simulink model "CM010C_GmG2kcaMcuCfg"  (R2013b)
settings: Solver=FixedStepDiscrete  SolverMode=SingleTasking  StartTime=0.0  StopTime=1  FixedStep=0.0005  RelTol=1e-3
values from neighbouring files (symbols this model uses):
  BATTVLTGSCAGFAC_ULS_F32 = DataDict.Constant    [CM010C_GmG2kcaMcuCfg_DataDict.m]
  BATTVLTGSWD1SCAGFAC_ULS_F32 = DataDict.Constant    [CM010C_GmG2kcaMcuCfg_DataDict.m]
undefined symbols (not defined in the file or in its folder): sigbuilder_block
libraries: CM010C_GmG2kcaMcuCfg_ModelLibrary x48, simulink x32
(part 1 of 2)
settings Model: Creator=nz3zln  LastModifiedBy=nz3zln
settings SolverCC: AutoInsertRateTranBlk=on  InsertRTBMode=Always
settings DataIOCC: LimitDataPoints=off  SaveFormat=Structure  ReturnWorkspaceOutputs=on
settings OptimizationCC: BlockReduction=off  InlineParams=on  ZeroExternalMemoryAtStartup=off  ZeroInternalMemoryAtStartup=off  OptimizeModelRefInitCode=on  LifeSpan=1
settings DebuggingCC: SignalInfNanChecking=error  SignalRangeChecking=warning  UnderspecifiedInitializationDetection=Simplified  SolverPrmCheckMsg=error  InheritedTsInSrcMsg=error  DiscreteInheritContinuousMsg=error  SingleTaskRateTransMsg=error  TasksWithSamePriorityMsg=error  SigSpecEnsureSampleTimeMsg=error  CheckMatrixSingularityMsg=error  ParameterUnderflowMsg=error  ParameterPrecisionLossMsg=error  ParameterTunabilityLossMsg=error  FixptConstUnderflowMsg=warning  FixptConstOverflowMsg=warning  VectorMatrixConversionMsg=error  SignalLabelMismatchMsg=error  UnconnectedInputMsg=error  UnconnectedOutputMsg=error  UnconnectedLineMsg=error  SFcnCompatibilityMsg=error  UniqueDataStoreMsg=warning  BusObjectLabelMismatch=error  RootOutportRequireBusObject=error  AssertControl=DisableAll  ModelReferenceIOMsg=error  ModelReferenceVersionMismatchMessage=warning  ModelReferenceIOMismatchMessage=error  ModelReferenceCSMismatchMessage=warning  ModelReferenceDataLoggingMessage=error  StateNameClashWarn=warning  StrictBusMsg=ErrorOnBusTreatedAsVector  NonBusSignalsTreatedAsBus=error  SFUnexpectedBacktrackingDiag=error  SFInvalidInputDataAccessInChartInitDiag=error  SFNoUnconditionalDefaultTransitionDiag=error  SFTransitionOutsideNaturalParentDiag=error  SFUnconditionalTransitionShadowingDiag=error  SFUndirectedBroadcastEventsDiag=error
settings ModelReferenceCC: ModelReferenceNumInstancesAllowed=Single
settings RTWCC: SystemTargetFile=autosar.tlc  GenCodeOnly=on  TemplateMakefile=ert_default_tmf  Description=AUTOSAR  GenerateReport=on  ProcessScript=autosar_make_rtw_hook  LaunchReport=on
settings CodeAppCC: GenerateComments=off  IgnoreCustomStorageClasses=off  CustomSymbolStrType=$N$R$M  CustomSymbolStrBlkIO=$N$M  SimulinkBlockComments=off
settings STFCustomTargetCC: ParMdlRefBuildCompliant=on  CompOptLevelCompliant=on  IncludeMdlTerminateFcn=off  CombineOutputUpdateFcns=on  SuppressErrorStatus=on  ERTFirstTimeCompliant=on  ERTCustomFileBanners=on  SupportNonFinite=off  SupportComplex=off  SupportContinuousTime=off  SupportNonInlinedSFcns=off  MATLABClassNameForMDSCustomization=Simulink.SoftwareTarget.ERTCustomization  AutosarCompliant=on  GRTInterface=off  SystemTargetFile=autosar.tlc
settings ERTTargetCC: CodeReplacementLibrary=ANSI_C  ConcurrentExecutionCompliant=off  IncludeMdlTerminateFcn=off  SuppressErrorStatus=on  SupportNonFinite=off  SupportComplex=off  ModelStepFunctionPrototypeControlCompliant=off  CPPClassGenCompliant=off  AutosarCompliant=on  InlinedParameterPlacement=NonHierarchical  ERTCustomFileTemplate=example_file_process.tlc  EnableUserReplacementTypes=on

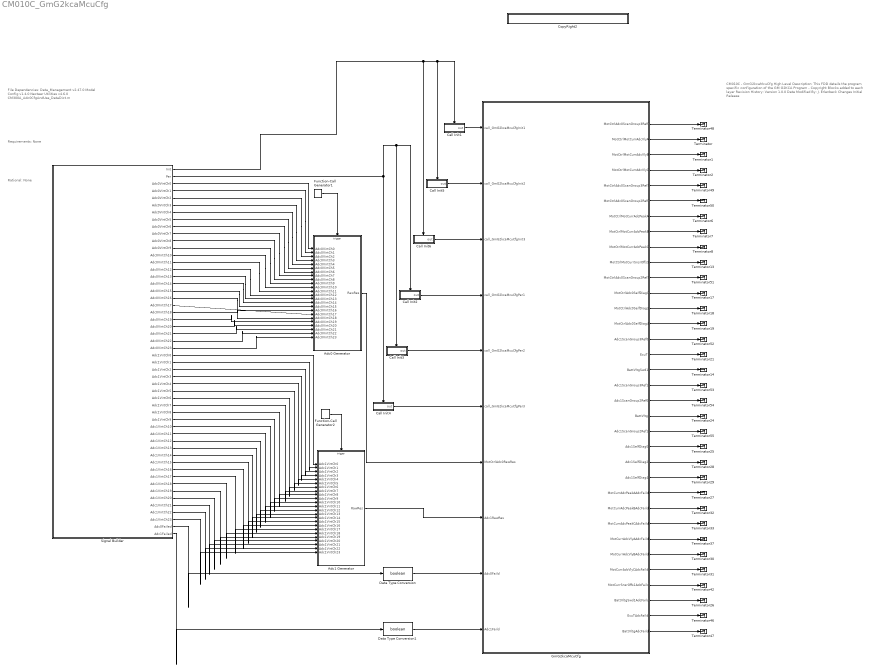
== system CM010C_GmG2kcaMcuCfg ==
  note: File Dependencies:
      |
      | Data_Management v2.47.0
      | Model Config v1.4.0
      | Nexteer Utilities v4.6.0
      | CM300A_Adc0CfgAndUse_DataDict.m
  note: CM010C - GmG2kcaMcuCfg
      |
      | High Level Description:
      | This FDD details the program specific configuration of the GM G2KCA Program
      |  - Copyright Blocks added to each layer
      |
      | Revision History:
      |
      | Version		1.0.0
      | Date
      | Modified By: 	J. Erlenbeck
      | Changes		Initial Release
  note: Requirements:
      |
      | None
  note: Rational:
      |
      | None
  Adc0 Generator : Subsystem  TreatAsAtomicUnit=on
  Adc1 Generator : Subsystem  TreatAsAtomicUnit=on
  Call Init1 : Subsystem  TreatAsAtomicUnit=on
  Call Init2 : Subsystem  TreatAsAtomicUnit=on
  Call Init3 : Subsystem  TreatAsAtomicUnit=on
  Call Init4 : Subsystem  TreatAsAtomicUnit=on
  Call Init5 : Subsystem  TreatAsAtomicUnit=on
  Call Init6 : Subsystem  TreatAsAtomicUnit=on
  CopyRight2 : Subsystem  Description=|  mask(Copyright Information){none=on}
      | Copyright info block.                                               
      |                                                                     
      | Place copyright information at the top of every subsystem in design.
      mask prompts: none "No parameters"
      mask help: Place copyright information at the top of every subsystem in design.
      mask Display:
      | NxtrConf = 'Nexteer Confidential';
      | 
      | sys = bdroot; %handle for the current model ("system")
      | first = get_param(sys,'Created');
      | first = first(end-3:end);  %year is last four digits
      | 
      | last = get_param(sys,'LastModifiedDate');
      | if isempty(last)
      |     last = datestr(now,'yyyy');
      | else
      |     last = last(end-3:end);
      | end
      | 
      | if strcmp(first,last)
      |     fprintf('%s -- Copyright %s Nexteer',NxtrConf,first)
      | else
      |     fprintf('%s -- %s%s- %s Nexteer',NxtrConf,char(169),first,last)
      | end
  Data Type Conversion : DataTypeConversion  OutDataTypeStr=boolean
  Data Type Conversion1 : DataTypeConversion  OutDataTypeStr=boolean
  Function-Call Generator1 : simulink/Ports & Subsystems/Function-Call Generator  sample_time=0.0005  numberOfIterations=1
  Function-Call Generator2 : simulink/Ports & Subsystems/Function-Call Generator  sample_time=0.0005  numberOfIterations=1
  GmG2kcaMcuCfg : Subsystem
  Signal Builder : Subsystem  Tag=STV Subsys  RequirementInfo={} %GIDa_2822100e_29fa_4197_9ccc_01864625f252  LoadFcn=sigbuilder_block('load');  StartFcn=sigbuilder_block('start');  StopFcn=sigbuilder_block('stop');  ClipboardFcn=sigbuilder_block('clipboard');  mask(Sigbuilder block){}
      mask help: Simulink:masks:SigbuilderBlock_MD
      mask init:
      | if ~strcmp(get_param(bdroot(gcbh),'SimulationStatus'),'stopped') tuvar = sigbuilder_block('maskInit'); end
      settings: CopyFcn=sigbuilder_block('copy');  DeleteFcn=sigbuilder_block('delete');  ModelCloseFcn=sigbuilder_block('modelClose');  PreSaveFcn=sigbuilder_block('preSave');  PauseFcn=sigbuilder_block('pause');  ContinueFcn=sigbuilder_block('continue');  NameChangeFcn=sigbuilder_block('namechange');  OpenFcn=sigbuilder_block('open',[6.2069 35.3793 1178.69 576 ]);  CloseFcn=sigbuilder_block('close');
      mask Display: plot(0, 0, 100, 100,[2, 2, 32, 32, 2], [68, 8, 8, 68, 68],[32, 2], [38, 38], [32, 19, 2],[53, 60, 44], [32, 17, 17, 2],[16, 16, 31, 31]);txt = getActiveGroup(gcbh);text(2, 100, txt,'verticalAlignment', 'top');
  Terminator{,1..2,6..8,13..14,17..19,21,24..33,37,42,46..55} (34 alike) : Terminator
  wires:
  Call Init1/1(out) -> GmG2kcaMcuCfg/1(call_GmG2kcaMcuCfgInit1)
  Call Init2/1(out) -> GmG2kcaMcuCfg/4(call_GmG2kcaMcuCfgPer1)
  Call Init3/1(out) -> GmG2kcaMcuCfg/5(call_GmG2kcaMcuCfgPer2)
  GmG2kcaMcuCfg/2(MotCtrlMotCurrAdcVlyA) -> Terminator/1
  GmG2kcaMcuCfg/3(MotCtrlMotCurrAdcVlyB) -> Terminator1/1
  GmG2kcaMcuCfg/4(MotCtrlMotCurrAdcVlyC) -> Terminator2/1
  GmG2kcaMcuCfg/7(MotCtrlMotCurrAdcPeakA) -> Terminator6/1
  GmG2kcaMcuCfg/8(MotCtrlMotCurrAdcPeakB) -> Terminator7/1
  GmG2kcaMcuCfg/9(MotCtrlMotCurrAdcPeakC) -> Terminator8/1
  GmG2kcaMcuCfg/10(MotCtrlMotCurrSnsrOffs1) -> Terminator13/1
  GmG2kcaMcuCfg/12(MotCtrlAdc0SelfDiag0) -> Terminator17/1
  GmG2kcaMcuCfg/13(MotCtrlAdc0SelfDiag2) -> Terminator18/1
  GmG2kcaMcuCfg/14(MotCtrlAdc0SelfDiag4) -> Terminator19/1
  GmG2kcaMcuCfg/16(EcuT) -> Terminator21/1
  GmG2kcaMcuCfg/17(BattVltgSwd1) -> Terminator14/1
  GmG2kcaMcuCfg/20(BattVltg) -> Terminator24/1
  GmG2kcaMcuCfg/22(Adc1SelfDiag0) -> Terminator25/1
  GmG2kcaMcuCfg/23(Adc1SelfDiag2) -> Terminator28/1
  GmG2kcaMcuCfg/24(Adc1SelfDiag4) -> Terminator29/1
  GmG2kcaMcuCfg/25(MotCurrAdcPeakAAdcFaild) -> Terminator27/1
  GmG2kcaMcuCfg/26(MotCurrAdcPeakBAdcFaild) -> Terminator32/1
  GmG2kcaMcuCfg/27(MotCurrAdcPeakCAdcFaild) -> Terminator33/1
  GmG2kcaMcuCfg/28(MotCurrAdcVlyAAdcFaild) -> Terminator37/1
  GmG2kcaMcuCfg/29(MotCurrAdcVlyBAdcFaild) -> Terminator30/1
  GmG2kcaMcuCfg/30(MotCurrAdcVlyCAdcFaild) -> Terminator31/1
  GmG2kcaMcuCfg/31(MotCurrSnsrOffs1AdcFaild) -> Terminator42/1
  GmG2kcaMcuCfg/32(BattVltgSwd1AdcFaild) -> Terminator26/1
  GmG2kcaMcuCfg/33(EcuTAdcFaild) -> Terminator46/1
  Call Init4/1(out) -> GmG2kcaMcuCfg/6(call_GmG2kcaMcuCfgPer3)
  Call Init5/1(out) -> GmG2kcaMcuCfg/2(call_GmG2kcaMcuCfgInit2)
  Call Init6/1(out) -> GmG2kcaMcuCfg/3(call_GmG2kcaMcuCfgInit3)
  GmG2kcaMcuCfg/34(BattVltgAdcFaild) -> Terminator47/1
  GmG2kcaMcuCfg/1(MotCtrlAdc0ScanGroup3Ref0) -> Terminator48/1
  GmG2kcaMcuCfg/5(MotCtrlAdc0ScanGroup3Ref1) -> Terminator49/1
  GmG2kcaMcuCfg/6(MotCtrlAdc0ScanGroup2Ref0) -> Terminator50/1
  GmG2kcaMcuCfg/11(MotCtrlAdc0ScanGroup2Ref1) -> Terminator51/1
  GmG2kcaMcuCfg/15(Adc1ScanGroup3Ref0) -> Terminator52/1
  GmG2kcaMcuCfg/18(Adc1ScanGroup3Ref1) -> Terminator53/1
  GmG2kcaMcuCfg/19(Adc1ScanGroup2Ref0) -> Terminator54/1
  GmG2kcaMcuCfg/21(Adc1ScanGroup2Ref1) -> Terminator55/1
  Function-Call Generator1/1 -> Adc0 Generator/Trigger
  Signal Builder/1(Init) -> Call Init6/Enable, Call Init5/Enable, Call Init1/Enable
  Signal Builder/2(Per) -> Call Init3/Enable, Call Init2/Enable, Call Init4/Enable
  Signal Builder/26(Adc0VirtCh23) -> Adc0 Generator/24(Adc0VirtCh23)
  Signal Builder/25(Adc0VirtCh22) -> Adc0 Generator/23(Adc0VirtCh22)
  Signal Builder/24(Adc0VirtCh21) -> Adc0 Generator/22(Adc0VirtCh21)
  Signal Builder/23(Adc0VirtCh20) -> Adc0 Generator/21(Adc0VirtCh20)
  Signal Builder/22(Adc0VirtCh19) -> Adc0 Generator/20(Adc0VirtCh19)
  Signal Builder/21(Adc0VirtCh18) -> Adc0 Generator/19(Adc0VirtCh18)
  Signal Builder/20(Adc0VirtCh17) -> Adc0 Generator/18(Adc0VirtCh17)
  Signal Builder/19(Adc0VirtCh16) -> Adc0 Generator/17(Adc0VirtCh16)
  Signal Builder/18(Adc0VirtCh15) -> Adc0 Generator/16(Adc0VirtCh15)
  Signal Builder/17(Adc0VirtCh14) -> Adc0 Generator/15(Adc0VirtCh14)
  Signal Builder/16(Adc0VirtCh13) -> Adc0 Generator/14(Adc0VirtCh13)
  Signal Builder/15(Adc0VirtCh12) -> Adc0 Generator/13(Adc0VirtCh12)
  Signal Builder/14(Adc0VirtCh11) -> Adc0 Generator/12(Adc0VirtCh11)
  Signal Builder/13(Adc0VirtCh10) -> Adc0 Generator/11(Adc0VirtCh10)
  Signal Builder/12(Adc0VirtCh9) -> Adc0 Generator/10(Adc0VirtCh9)
  Signal Builder/11(Adc0VirtCh8) -> Adc0 Generator/9(Adc0VirtCh8)
  Signal Builder/10(Adc0VirtCh7) -> Adc0 Generator/8(Adc0VirtCh7)
  Signal Builder/9(Adc0VirtCh6) -> Adc0 Generator/7(Adc0VirtCh6)
  Signal Builder/8(Adc0VirtCh5) -> Adc0 Generator/6(Adc0VirtCh5)
  Signal Builder/7(Adc0VirtCh4) -> Adc0 Generator/5(Adc0VirtCh4)
  Signal Builder/6(Adc0VirtCh3) -> Adc0 Generator/4(Adc0VirtCh3)
  Signal Builder/5(Adc0VirtCh2) -> Adc0 Generator/3(Adc0VirtCh2)
  Signal Builder/4(Adc0VirtCh1) -> Adc0 Generator/2(Adc0VirtCh1)
  Signal Builder/3(Adc0VirtCh0) -> Adc0 Generator/1(Adc0VirtCh0)
  Adc0 Generator/1(RawRes) -> GmG2kcaMcuCfg/7(MotCtrlAdc0RawRes)
  Signal Builder/50(Adc1VirtCh23) -> Adc1 Generator/24(Adc1VirtCh23)
  Signal Builder/49(Adc1VirtCh22) -> Adc1 Generator/23(Adc1VirtCh22)
  Signal Builder/48(Adc1VirtCh21) -> Adc1 Generator/22(Adc1VirtCh21)
  Signal Builder/47(Adc1VirtCh20) -> Adc1 Generator/21(Adc1VirtCh20)
  Signal Builder/46(Adc1VirtCh19) -> Adc1 Generator/20(Adc1VirtCh19)
  Signal Builder/45(Adc1VirtCh18) -> Adc1 Generator/19(Adc1VirtCh18)
  Signal Builder/44(Adc1VirtCh17) -> Adc1 Generator/18(Adc1VirtCh17)
  Signal Builder/43(Adc1VirtCh16) -> Adc1 Generator/17(Adc1VirtCh16)
  Signal Builder/42(Adc1VirtCh15) -> Adc1 Generator/16(Adc1VirtCh15)
  Signal Builder/41(Adc1VirtCh14) -> Adc1 Generator/15(Adc1VirtCh14)
  Signal Builder/40(Adc1VirtCh13) -> Adc1 Generator/14(Adc1VirtCh13)
  Signal Builder/39(Adc1VirtCh12) -> Adc1 Generator/13(Adc1VirtCh12)
  Signal Builder/38(Adc1VirtCh11) -> Adc1 Generator/12(Adc1VirtCh11)
  Signal Builder/37(Adc1VirtCh10) -> Adc1 Generator/11(Adc1VirtCh10)
  Signal Builder/36(Adc1VirtCh9) -> Adc1 Generator/10(Adc1VirtCh9)
  Signal Builder/35(Adc1VirtCh8) -> Adc1 Generator/9(Adc1VirtCh8)
  Signal Builder/34(Adc1VirtCh7) -> Adc1 Generator/8(Adc1VirtCh7)
  Signal Builder/33(Adc1VirtCh6) -> Adc1 Generator/7(Adc1VirtCh6)
  Signal Builder/32(Adc1VirtCh5) -> Adc1 Generator/6(Adc1VirtCh5)
  Signal Builder/31(Adc1VirtCh4) -> Adc1 Generator/5(Adc1VirtCh4)
  Signal Builder/30(Adc1VirtCh3) -> Adc1 Generator/4(Adc1VirtCh3)
  Signal Builder/29(Adc1VirtCh2) -> Adc1 Generator/3(Adc1VirtCh2)
  Signal Builder/28(Adc1VirtCh1) -> Adc1 Generator/2(Adc1VirtCh1)
  Signal Builder/27(Adc1VirtCh0) -> Adc1 Generator/1(Adc1VirtCh0)
  Function-Call Generator2/1 -> Adc1 Generator/Trigger
  Adc1 Generator/1(RawRes) -> GmG2kcaMcuCfg/8(Adc1RawRes)
  Signal Builder/51(Adc0Failed) -> Data Type Conversion/1
  Signal Builder/52(Adc1Failed) -> Data Type Conversion1/1
  Data Type Conversion/1 -> GmG2kcaMcuCfg/9(Adc0Faild)
  Data Type Conversion1/1 -> GmG2kcaMcuCfg/10(Adc1Faild)

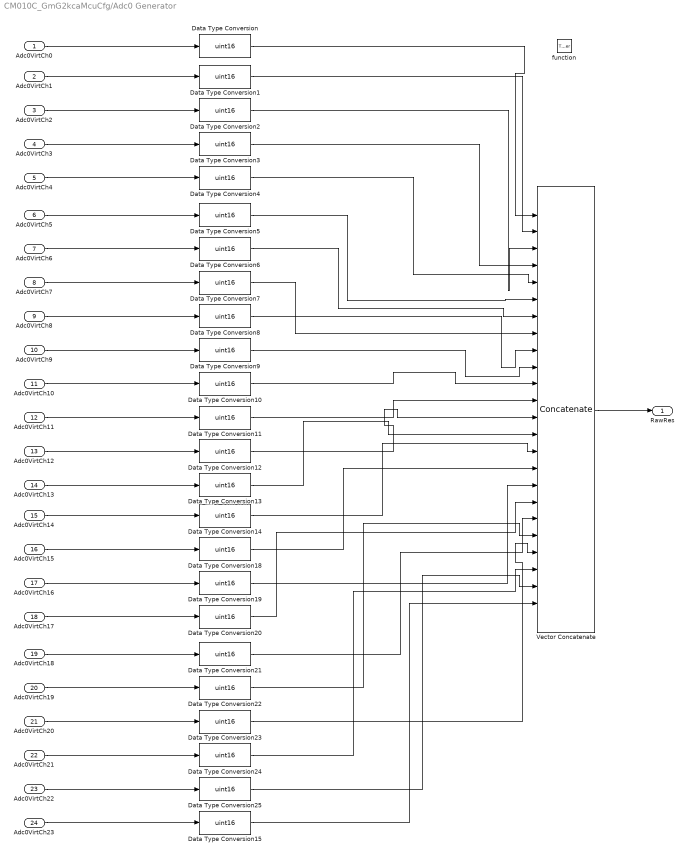
== system CM010C_GmG2kcaMcuCfg/Adc0 Generator ==
  Adc0VirtCh0 : Inport
  Adc0VirtCh1 : Inport  Port=2
  Adc0VirtCh2 : Inport  Port=3
  Adc0VirtCh3 : Inport  Port=4
  Adc0VirtCh4 : Inport  Port=5
  Adc0VirtCh5 : Inport  Port=6
  Adc0VirtCh6 : Inport  Port=7
  Adc0VirtCh7 : Inport  Port=8
  Adc0VirtCh8 : Inport  Port=9
  Adc0VirtCh9 : Inport  Port=10
  Adc0VirtCh10 : Inport  Port=11
  Adc0VirtCh11 : Inport  Port=12
  Adc0VirtCh12 : Inport  Port=13
  Adc0VirtCh13 : Inport  Port=14
  Adc0VirtCh14 : Inport  Port=15
  Adc0VirtCh15 : Inport  Port=16
  Adc0VirtCh16 : Inport  Port=17
  Adc0VirtCh17 : Inport  Port=18
  Adc0VirtCh18 : Inport  Port=19
  Adc0VirtCh19 : Inport  Port=20
  Adc0VirtCh20 : Inport  Port=21
  Adc0VirtCh21 : Inport  Port=22
  Adc0VirtCh22 : Inport  Port=23
  Adc0VirtCh23 : Inport  Port=24
  function : TriggerPort  TriggerType=function-call
  Data Type Conversion{,1..15,18..25} (24 alike) : DataTypeConversion  OutDataTypeStr=uint16
  Vector Concatenate : Concatenate  NumInputs=24
  RawRes : Outport
  wires:
  Adc0VirtCh0/1 -> Data Type Conversion/1
  Data Type Conversion/1 -> Vector Concatenate/1
  Adc0VirtCh1/1 -> Data Type Conversion1/1
  Adc0VirtCh2/1 -> Data Type Conversion2/1
  Adc0VirtCh3/1 -> Data Type Conversion3/1
  Adc0VirtCh4/1 -> Data Type Conversion4/1
  Adc0VirtCh5/1 -> Data Type Conversion5/1
  Adc0VirtCh6/1 -> Data Type Conversion6/1
  Adc0VirtCh7/1 -> Data Type Conversion7/1
  Adc0VirtCh8/1 -> Data Type Conversion8/1
  Adc0VirtCh9/1 -> Data Type Conversion9/1
  Adc0VirtCh10/1 -> Data Type Conversion10/1
  Adc0VirtCh11/1 -> Data Type Conversion11/1
  Adc0VirtCh12/1 -> Data Type Conversion12/1
  Adc0VirtCh13/1 -> Data Type Conversion13/1
  Adc0VirtCh14/1 -> Data Type Conversion14/1
  Adc0VirtCh15/1 -> Data Type Conversion18/1
  Adc0VirtCh17/1 -> Data Type Conversion20/1
  Adc0VirtCh18/1 -> Data Type Conversion21/1
  Adc0VirtCh19/1 -> Data Type Conversion22/1
  Adc0VirtCh20/1 -> Data Type Conversion23/1
  Adc0VirtCh21/1 -> Data Type Conversion24/1
  Adc0VirtCh23/1 -> Data Type Conversion15/1
  Adc0VirtCh16/1 -> Data Type Conversion19/1
  Adc0VirtCh22/1 -> Data Type Conversion25/1
  Data Type Conversion1/1 -> Vector Concatenate/2
  Data Type Conversion2/1 -> Vector Concatenate/3
  Data Type Conversion3/1 -> Vector Concatenate/4
  Data Type Conversion4/1 -> Vector Concatenate/5
  Data Type Conversion5/1 -> Vector Concatenate/6
  Data Type Conversion6/1 -> Vector Concatenate/7
  Data Type Conversion7/1 -> Vector Concatenate/8
  Data Type Conversion8/1 -> Vector Concatenate/9
  Data Type Conversion9/1 -> Vector Concatenate/10
  Data Type Conversion10/1 -> Vector Concatenate/11
  Data Type Conversion11/1 -> Vector Concatenate/12
  Data Type Conversion12/1 -> Vector Concatenate/13
  Data Type Conversion13/1 -> Vector Concatenate/14
  Data Type Conversion14/1 -> Vector Concatenate/15
  Data Type Conversion18/1 -> Vector Concatenate/16
  Data Type Conversion19/1 -> Vector Concatenate/17
  Data Type Conversion20/1 -> Vector Concatenate/18
  Data Type Conversion21/1 -> Vector Concatenate/19
  Data Type Conversion22/1 -> Vector Concatenate/20
  Data Type Conversion23/1 -> Vector Concatenate/21
  Data Type Conversion24/1 -> Vector Concatenate/22
  Data Type Conversion25/1 -> Vector Concatenate/23
  Data Type Conversion15/1 -> Vector Concatenate/24
  Vector Concatenate/1 -> RawRes/1

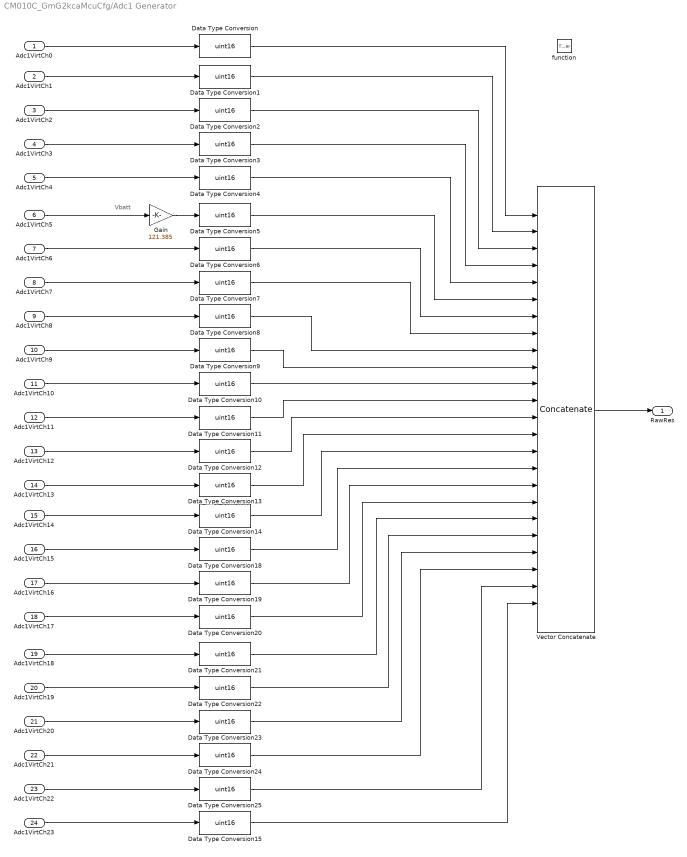
== system CM010C_GmG2kcaMcuCfg/Adc1 Generator ==
  note: Vbatt
  Adc1VirtCh0 : Inport
  Adc1VirtCh1 : Inport  Port=2
  Adc1VirtCh2 : Inport  Port=3
  Adc1VirtCh3 : Inport  Port=4
  Adc1VirtCh4 : Inport  Port=5
  Adc1VirtCh5 : Inport  Port=6
  Adc1VirtCh6 : Inport  Port=7
  Adc1VirtCh7 : Inport  Port=8
  Adc1VirtCh8 : Inport  Port=9
  Adc1VirtCh9 : Inport  Port=10
  Adc1VirtCh10 : Inport  Port=11
  Adc1VirtCh11 : Inport  Port=12
  Adc1VirtCh12 : Inport  Port=13
  Adc1VirtCh13 : Inport  Port=14
  Adc1VirtCh14 : Inport  Port=15
  Adc1VirtCh15 : Inport  Port=16
  Adc1VirtCh16 : Inport  Port=17
  Adc1VirtCh17 : Inport  Port=18
  Adc1VirtCh18 : Inport  Port=19
  Adc1VirtCh19 : Inport  Port=20
  Adc1VirtCh20 : Inport  Port=21
  Adc1VirtCh21 : Inport  Port=22
  Adc1VirtCh22 : Inport  Port=23
  Adc1VirtCh23 : Inport  Port=24
  function : TriggerPort  TriggerType=function-call
  Data Type Conversion{,1..15,18..25} (24 alike) : DataTypeConversion  OutDataTypeStr=uint16
  Gain : Gain  Gain=121.385
  Vector Concatenate : Concatenate  NumInputs=24
  RawRes : Outport
  wires:
  Vector Concatenate/1 -> RawRes/1
  Data Type Conversion15/1 -> Vector Concatenate/24
  Data Type Conversion25/1 -> Vector Concatenate/23
  Data Type Conversion24/1 -> Vector Concatenate/22
  Data Type Conversion23/1 -> Vector Concatenate/21
  Data Type Conversion22/1 -> Vector Concatenate/20
  Data Type Conversion21/1 -> Vector Concatenate/19
  Data Type Conversion20/1 -> Vector Concatenate/18
  Data Type Conversion19/1 -> Vector Concatenate/17
  Data Type Conversion18/1 -> Vector Concatenate/16
  Data Type Conversion14/1 -> Vector Concatenate/15
  Data Type Conversion13/1 -> Vector Concatenate/14
  Data Type Conversion12/1 -> Vector Concatenate/13
  Data Type Conversion11/1 -> Vector Concatenate/12
  Data Type Conversion10/1 -> Vector Concatenate/11
  Data Type Conversion9/1 -> Vector Concatenate/10
  Data Type Conversion8/1 -> Vector Concatenate/9
  Data Type Conversion7/1 -> Vector Concatenate/8
  Data Type Conversion6/1 -> Vector Concatenate/7
  Data Type Conversion5/1 -> Vector Concatenate/6
  Data Type Conversion4/1 -> Vector Concatenate/5
  Data Type Conversion3/1 -> Vector Concatenate/4
  Data Type Conversion2/1 -> Vector Concatenate/3
  Data Type Conversion1/1 -> Vector Concatenate/2
  Adc1VirtCh22/1 -> Data Type Conversion25/1
  Adc1VirtCh16/1 -> Data Type Conversion19/1
  Adc1VirtCh23/1 -> Data Type Conversion15/1
  Adc1VirtCh21/1 -> Data Type Conversion24/1
  Adc1VirtCh20/1 -> Data Type Conversion23/1
  Adc1VirtCh19/1 -> Data Type Conversion22/1
  Adc1VirtCh18/1 -> Data Type Conversion21/1
  Adc1VirtCh17/1 -> Data Type Conversion20/1
  Adc1VirtCh15/1 -> Data Type Conversion18/1
  Adc1VirtCh14/1 -> Data Type Conversion14/1
  Adc1VirtCh13/1 -> Data Type Conversion13/1
  Adc1VirtCh12/1 -> Data Type Conversion12/1
  Adc1VirtCh11/1 -> Data Type Conversion11/1
  Adc1VirtCh10/1 -> Data Type Conversion10/1
  Adc1VirtCh9/1 -> Data Type Conversion9/1
  Adc1VirtCh8/1 -> Data Type Conversion8/1
  Adc1VirtCh7/1 -> Data Type Conversion7/1
  Adc1VirtCh6/1 -> Data Type Conversion6/1
  Adc1VirtCh5/1 -> Gain/1
  Adc1VirtCh4/1 -> Data Type Conversion4/1
  Adc1VirtCh3/1 -> Data Type Conversion3/1
  Adc1VirtCh2/1 -> Data Type Conversion2/1
  Adc1VirtCh1/1 -> Data Type Conversion1/1
  Data Type Conversion/1 -> Vector Concatenate/1
  Adc1VirtCh0/1 -> Data Type Conversion/1
  Gain/1 -> Data Type Conversion5/1

== system CM010C_GmG2kcaMcuCfg/Call Init1 ==
  Enable : EnablePort
  Function Call Trigger : simulink/Ports & Subsystems/Function-Call Generator  RequirementInfo="{'linktype_rmi_doors' '000089e3 (/E-STEER_New/System Specification Documents/Core Specs/Subsystem Specs/System Functions FDD/SF-46  Gross Cross Check)' '#211' 'true' '3.1-1 The GCC function shall monitor every posted output motor comm' '' ; 'linktype_rmi_doors' '000089e3 (/E-STEER_New/System Specification Documents/Core Specs/Subsystem Specs/System Functions FDD/SF-46  Gross Cross Check)' '#182' 'true' '3.2.2-1 GCC shall be executed at a 0.002 second loop time.' '' } %GIDa_ff755a2e_49d1_45f7_8591_3ce0ef475338"  sample_time=0.0005  numberOfIterations=1
  out : Outport
  wires:
  Function Call Trigger/1 -> out/1

== system CM010C_GmG2kcaMcuCfg/Call Init2 ==
  Enable : EnablePort
  Function Call Trigger : simulink/Ports & Subsystems/Function-Call Generator  RequirementInfo="{'linktype_rmi_doors' '000089e3 (/E-STEER_New/System Specification Documents/Core Specs/Subsystem Specs/System Functions FDD/SF-46  Gross Cross Check)' '#211' 'true' '3.1-1 The GCC function shall monitor every posted output motor comm' '' ; 'linktype_rmi_doors' '000089e3 (/E-STEER_New/System Specification Documents/Core Specs/Subsystem Specs/System Functions FDD/SF-46  Gross Cross Check)' '#182' 'true' '3.2.2-1 GCC shall be executed at a 0.002 second loop time.' '' } %GIDa_ba5be832_aeac_40ae_ae53_3fd25198366e"  sample_time=0.0005  numberOfIterations=1
  out : Outport
  wires:
  Function Call Trigger/1 -> out/1

== system CM010C_GmG2kcaMcuCfg/Call Init3 ==
  Enable : EnablePort
  Function Call Trigger : simulink/Ports & Subsystems/Function-Call Generator  RequirementInfo="{'linktype_rmi_doors' '000089e3 (/E-STEER_New/System Specification Documents/Core Specs/Subsystem Specs/System Functions FDD/SF-46  Gross Cross Check)' '#211' 'true' '3.1-1 The GCC function shall monitor every posted output motor comm' '' ; 'linktype_rmi_doors' '000089e3 (/E-STEER_New/System Specification Documents/Core Specs/Subsystem Specs/System Functions FDD/SF-46  Gross Cross Check)' '#182' 'true' '3.2.2-1 GCC shall be executed at a 0.002 second loop time.' '' } %GIDa_bf682727_f4b1_4f52_ae72_c6f6d8d412d7"  sample_time=0.002  numberOfIterations=1
  out : Outport
  wires:
  Function Call Trigger/1 -> out/1

== system CM010C_GmG2kcaMcuCfg/Call Init4 ==
  Enable : EnablePort
  Function Call Trigger : simulink/Ports & Subsystems/Function-Call Generator  RequirementInfo="{'linktype_rmi_doors' '000089e3 (/E-STEER_New/System Specification Documents/Core Specs/Subsystem Specs/System Functions FDD/SF-46  Gross Cross Check)' '#211' 'true' '3.1-1 The GCC function shall monitor every posted output motor comm' '' ; 'linktype_rmi_doors' '000089e3 (/E-STEER_New/System Specification Documents/Core Specs/Subsystem Specs/System Functions FDD/SF-46  Gross Cross Check)' '#182' 'true' '3.2.2-1 GCC shall be executed at a 0.002 second loop time.' '' } %GIDa_39162fcb_260a_4191_9640_bf2fa4fe87e2"  sample_time=0.002  numberOfIterations=1
  out : Outport
  wires:
  Function Call Trigger/1 -> out/1

== system CM010C_GmG2kcaMcuCfg/Call Init5 ==
  Enable : EnablePort
  Function Call Trigger : simulink/Ports & Subsystems/Function-Call Generator  RequirementInfo="{'linktype_rmi_doors' '000089e3 (/E-STEER_New/System Specification Documents/Core Specs/Subsystem Specs/System Functions FDD/SF-46  Gross Cross Check)' '#211' 'true' '3.1-1 The GCC function shall monitor every posted output motor comm' '' ; 'linktype_rmi_doors' '000089e3 (/E-STEER_New/System Specification Documents/Core Specs/Subsystem Specs/System Functions FDD/SF-46  Gross Cross Check)' '#182' 'true' '3.2.2-1 GCC shall be executed at a 0.002 second loop time.' '' } %GIDa_52b82f2d_d21e_4ccf_9b87_2b660c433421"  sample_time=0.0005  numberOfIterations=1
  out : Outport
  wires:
  Function Call Trigger/1 -> out/1

== system CM010C_GmG2kcaMcuCfg/Call Init6 ==
  Enable : EnablePort
  Function Call Trigger : simulink/Ports & Subsystems/Function-Call Generator  RequirementInfo="{'linktype_rmi_doors' '000089e3 (/E-STEER_New/System Specification Documents/Core Specs/Subsystem Specs/System Functions FDD/SF-46  Gross Cross Check)' '#211' 'true' '3.1-1 The GCC function shall monitor every posted output motor comm' '' ; 'linktype_rmi_doors' '000089e3 (/E-STEER_New/System Specification Documents/Core Specs/Subsystem Specs/System Functions FDD/SF-46  Gross Cross Check)' '#182' 'true' '3.2.2-1 GCC shall be executed at a 0.002 second loop time.' '' } %GIDa_40b20fc1_ef82_4ce8_9bb2_77ecb7477d85"  sample_time=0.002  numberOfIterations=1
  out : Outport
  wires:
  Function Call Trigger/1 -> out/1

== system CM010C_GmG2kcaMcuCfg/CopyRight2 ==

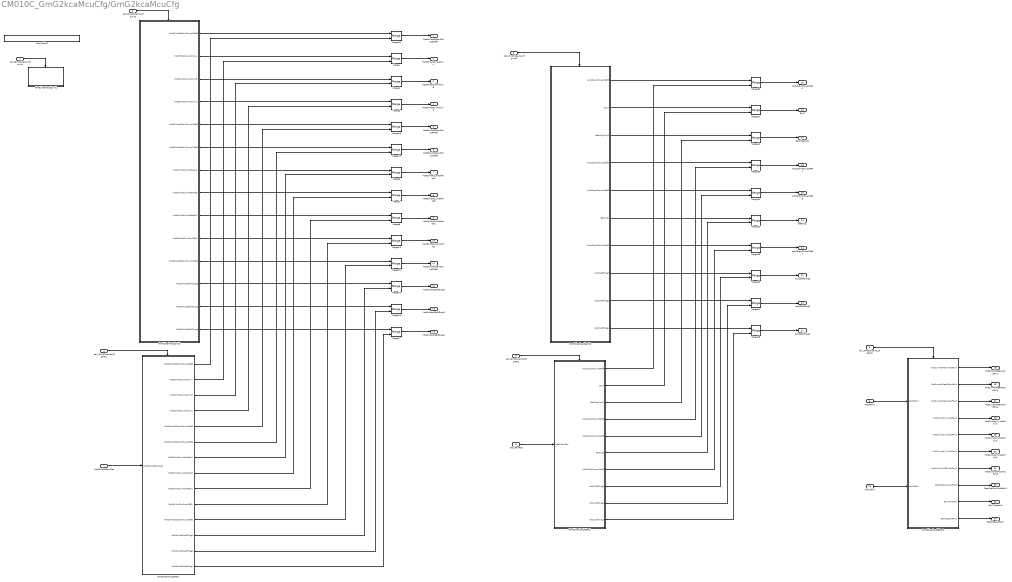
== system CM010C_GmG2kcaMcuCfg/GmG2kcaMcuCfg ==
  call_GmG2kcaMcuCfgInit1 : Inport
  call_GmG2kcaMcuCfgInit2 : Inport  Port=2
  call_GmG2kcaMcuCfgInit3 : Inport  Port=3
  call_GmG2kcaMcuCfgPer1 : Inport  Port=4
  call_GmG2kcaMcuCfgPer2 : Inport  Port=5
  call_GmG2kcaMcuCfgPer3 : Inport  Port=6
  MotCtrlAdc0RawRes : Inport  Port=7
  Adc1RawRes : Inport  Port=8
  Adc0Faild : Inport  Port=9
  Adc1Faild : Inport  Port=10
  CopyRight2 : Subsystem  Description=|  mask(Copyright Information){none=on}
      | Copyright info block.                                               
      |                                                                     
      | Place copyright information at the top of every subsystem in design.
      mask prompts: none "No parameters"
      mask help: Place copyright information at the top of every subsystem in design.
      mask Display:
      | NxtrConf = 'Nexteer Confidential';
      | 
      | sys = bdroot; %handle for the current model ("system")
      | first = get_param(sys,'Created');
      | first = first(end-3:end);  %year is last four digits
      | 
      | last = get_param(sys,'LastModifiedDate');
      | if isempty(last)
      |     last = datestr(now,'yyyy');
      | else
      |     last = last(end-3:end);
      | end
      | 
      | if strcmp(first,last)
      |     fprintf('%s -- Copyright %s Nexteer',NxtrConf,first)
      | else
      |     fprintf('%s -- %s%s- %s Nexteer',NxtrConf,char(169),first,last)
      | end
  GmG2kcaMcuCfgInit1 : Subsystem
  GmG2kcaMcuCfgInit2 : Subsystem
  GmG2kcaMcuCfgInit3 : Subsystem
  GmG2kcaMcuCfgPer1 : Subsystem  RequirementInfo={} %GIDa_cb8aed4e_f73b_4f5e_bbba_e7bbcee4a2fc
      settings: AttributesFormatString=Priority: %<Priority>
  GmG2kcaMcuCfgPer2 : Subsystem  RequirementInfo={} %GIDa_f8eec309_27b4_4df0_b18c_c2951f94362c
      settings: AttributesFormatString=Priority: %<Priority>
  GmG2kcaMcuCfgPer3 : Subsystem  RequirementInfo={} %GIDa_f61b09d0_e9f4_4379_bee3_c878705b543d
      settings: AttributesFormatString=Priority: %<Priority>
  Merge{,1..2,6..8,13,15..17,20,22..25,27..35} (24 alike) : Merge
  MotCtrlAdc0ScanGroup3Ref0 : Outport
  MotCtrlMotCurrAdcVlyA : Outport  Port=2
  MotCtrlMotCurrAdcVlyB : Outport  Port=3
  MotCtrlMotCurrAdcVlyC : Outport  Port=4
  MotCtrlAdc0ScanGroup3Ref1 : Outport  Port=5
  MotCtrlAdc0ScanGroup2Ref0 : Outport  Port=6
  MotCtrlMotCurrAdcPeakA : Outport  Port=7
  MotCtrlMotCurrAdcPeakB : Outport  Port=8
  MotCtrlMotCurrAdcPeakC : Outport  Port=9
  MotCtrlMotCurrSnsrOffs1 : Outport  Port=10
  MotCtrlAdc0ScanGroup2Ref1 : Outport  Port=11
  MotCtrlAdc0SelfDiag0 : Outport  Port=12
  MotCtrlAdc0SelfDiag2 : Outport  Port=13
  MotCtrlAdc0SelfDiag4 : Outport  Port=14
  Adc1ScanGroup3Ref0 : Outport  Port=15
  EcuT : Outport  Port=16
  BattVltgSwd1 : Outport  Port=17
  Adc1ScanGroup3Ref1 : Outport  Port=18
  Adc1ScanGroup2Ref0 : Outport  Port=19
  BattVltg : Outport  Port=20
  Adc1ScanGroup2Ref1 : Outport  Port=21
  Adc1SelfDiag0 : Outport  Port=22
  Adc1SelfDiag2 : Outport  Port=23
  Adc1SelfDiag4 : Outport  Port=24
  MotCurrAdcPeakAAdcFaild : Outport  Port=25
  MotCurrAdcPeakBAdcFaild : Outport  Port=26
  MotCurrAdcPeakCAdcFaild : Outport  Port=27
  MotCurrAdcVlyAAdcFaild : Outport  Port=28
  MotCurrAdcVlyBAdcFaild : Outport  Port=29
  MotCurrAdcVlyCAdcFaild : Outport  Port=30
  MotCurrSnsrOffs1AdcFaild : Outport  Port=31
  BattVltgSwd1AdcFaild : Outport  Port=32
  EcuTAdcFaild : Outport  Port=33
  BattVltgAdcFaild : Outport  Port=34
  wires:
  call_GmG2kcaMcuCfgPer1/1 -> GmG2kcaMcuCfgPer1/Trigger
  call_GmG2kcaMcuCfgPer2/1 -> GmG2kcaMcuCfgPer2/Trigger
  GmG2kcaMcuCfgInit2/2(MotCtrlMotCurrAdcVlyA) -> Merge/1
  Merge/1 -> MotCtrlMotCurrAdcVlyA/1
  GmG2kcaMcuCfgInit2/3(MotCtrlMotCurrAdcVlyB) -> Merge1/1
  Merge1/1 -> MotCtrlMotCurrAdcVlyB/1
  Merge2/1 -> MotCtrlMotCurrAdcVlyC/1
  GmG2kcaMcuCfgInit2/4(MotCtrlMotCurrAdcVlyC) -> Merge2/1
  GmG2kcaMcuCfgInit2/7(MotCtrlMotCurrAdcPeakA) -> Merge6/1
  Merge6/1 -> MotCtrlMotCurrAdcPeakA/1
  GmG2kcaMcuCfgInit2/8(MotCtrlMotCurrAdcPeakB) -> Merge7/1
  GmG2kcaMcuCfgInit2/9(MotCtrlMotCurrAdcPeakC) -> Merge8/1
  GmG2kcaMcuCfgInit2/10(MotCtrlMotCurrSnsrOffs1) -> Merge13/1
  Merge7/1 -> MotCtrlMotCurrAdcPeakB/1
  Merge8/1 -> MotCtrlMotCurrAdcPeakC/1
  Merge13/1 -> MotCtrlMotCurrSnsrOffs1/1
  GmG2kcaMcuCfgInit2/12(MotCtrlAdc0SelfDiag0) -> Merge15/1
  GmG2kcaMcuCfgInit2/13(MotCtrlAdc0SelfDiag2) -> Merge16/1
  GmG2kcaMcuCfgInit2/14(MotCtrlAdc0SelfDiag4) -> Merge17/1
  Merge15/1 -> MotCtrlAdc0SelfDiag0/1
  Merge16/1 -> MotCtrlAdc0SelfDiag2/1
  Merge17/1 -> MotCtrlAdc0SelfDiag4/1
  Merge27/1 -> EcuT/1
  Merge20/1 -> BattVltgSwd1/1
  Merge22/1 -> BattVltg/1
  Merge23/1 -> Adc1SelfDiag0/1
  Merge24/1 -> Adc1SelfDiag2/1
  Merge25/1 -> Adc1SelfDiag4/1
  GmG2kcaMcuCfgPer1/2(MotCtrlMotCurrAdcVlyA) -> Merge/2
  GmG2kcaMcuCfgPer1/3(MotCtrlMotCurrAdcVlyB) -> Merge1/2
  GmG2kcaMcuCfgPer1/4(MotCtrlMotCurrAdcVlyC) -> Merge2/2
  GmG2kcaMcuCfgPer1/7(MotCtrlMotCurrAdcPeakA) -> Merge6/2
  GmG2kcaMcuCfgPer1/8(MotCtrlMotCurrAdcPeakB) -> Merge7/2
  GmG2kcaMcuCfgPer1/9(MotCtrlMotCurrAdcPeakC) -> Merge8/2
  GmG2kcaMcuCfgPer1/10(MotCtrlMotCurrSnsrOffs1) -> Merge13/2
  GmG2kcaMcuCfgPer1/12(MotCtrlAdc0SelfDiag0) -> Merge15/2
  GmG2kcaMcuCfgPer1/13(MotCtrlAdc0SelfDiag2) -> Merge16/2
  GmG2kcaMcuCfgPer1/14(MotCtrlAdc0SelfDiag4) -> Merge17/2
  call_GmG2kcaMcuCfgInit1/1 -> GmG2kcaMcuCfgInit1/Trigger
  GmG2kcaMcuCfgInit3/2(EcuT) -> Merge27/1
  GmG2kcaMcuCfgInit3/3(BattVltgSwd1) -> Merge20/1
  GmG2kcaMcuCfgInit3/6(BattVltg) -> Merge22/1
  GmG2kcaMcuCfgInit3/8(Adc1SelfDiag0) -> Merge23/1
  GmG2kcaMcuCfgInit3/9(Adc1SelfDiag2) -> Merge24/1
  GmG2kcaMcuCfgInit3/10(Adc1SelfDiag4) -> Merge25/1
  GmG2kcaMcuCfgPer2/2(EcuT) -> Merge27/2
  GmG2kcaMcuCfgPer2/3(BattVltgSwd1) -> Merge20/2
  GmG2kcaMcuCfgPer2/6(BattVltg) -> Merge22/2
  GmG2kcaMcuCfgPer2/8(Adc1SelfDiag0) -> Merge23/2
  GmG2kcaMcuCfgPer2/9(Adc1SelfDiag2) -> Merge24/2
  GmG2kcaMcuCfgPer2/10(Adc1SelfDiag4) -> Merge25/2
  MotCtrlAdc0RawRes/1 -> GmG2kcaMcuCfgPer1/1(MotCtrlAdc0RawRes)
  Adc1RawRes/1 -> GmG2kcaMcuCfgPer2/1(Adc1RawRes)
  call_GmG2kcaMcuCfgPer3/1 -> GmG2kcaMcuCfgPer3/Trigger
  Adc0Faild/1 -> GmG2kcaMcuCfgPer3/1(Adc0Faild)
  Adc1Faild/1 -> GmG2kcaMcuCfgPer3/2(Adc1Faild)
  GmG2kcaMcuCfgPer3/1(MotCurrAdcPeakAAdcFaild) -> MotCurrAdcPeakAAdcFaild/1
  GmG2kcaMcuCfgPer3/2(MotCurrAdcPeakBAdcFaild) -> MotCurrAdcPeakBAdcFaild/1
  GmG2kcaMcuCfgPer3/3(MotCurrAdcPeakCAdcFaild) -> MotCurrAdcPeakCAdcFaild/1
  GmG2kcaMcuCfgPer3/4(MotCurrAdcVlyAAdcFaild) -> MotCurrAdcVlyAAdcFaild/1
  GmG2kcaMcuCfgPer3/5(MotCurrAdcVlyBAdcFaild) -> MotCurrAdcVlyBAdcFaild/1
  GmG2kcaMcuCfgPer3/6(MotCurrAdcVlyCAdcFaild) -> MotCurrAdcVlyCAdcFaild/1
  GmG2kcaMcuCfgPer3/7(MotCurrSnsrOffs1AdcFaild) -> MotCurrSnsrOffs1AdcFaild/1
  GmG2kcaMcuCfgPer3/8(BattVltgSwd1AdcFaild) -> BattVltgSwd1AdcFaild/1
  GmG2kcaMcuCfgPer3/9(EcuTAdcFaild) -> EcuTAdcFaild/1
  call_GmG2kcaMcuCfgInit2/1 -> GmG2kcaMcuCfgInit2/Trigger
  call_GmG2kcaMcuCfgInit3/1 -> GmG2kcaMcuCfgInit3/Trigger
  GmG2kcaMcuCfgPer3/10(BattVltgAdcFaild) -> BattVltgAdcFaild/1
  Merge28/1 -> MotCtrlAdc0ScanGroup3Ref1/1
  Merge29/1 -> MotCtrlAdc0ScanGroup2Ref0/1
  GmG2kcaMcuCfgInit2/5(MotCtrlAdc0ScanGroup3Ref1) -> Merge28/1
  GmG2kcaMcuCfgInit2/6(MotCtrlAdc0ScanGroup2Ref0) -> Merge29/1
  Merge30/1 -> MotCtrlAdc0ScanGroup3Ref0/1
  GmG2kcaMcuCfgInit2/1(MotCtrlAdc0ScanGroup3Ref0) -> Merge30/1
  Merge31/1 -> MotCtrlAdc0ScanGroup2Ref1/1
  GmG2kcaMcuCfgInit2/11(MotCtrlAdc0ScanGroup2Ref1) -> Merge31/1
  GmG2kcaMcuCfgPer1/1(MotCtrlAdc0ScanGroup3Ref0) -> Merge30/2
  GmG2kcaMcuCfgPer1/5(MotCtrlAdc0ScanGroup3Ref1) -> Merge28/2
  GmG2kcaMcuCfgPer1/6(MotCtrlAdc0ScanGroup2Ref0) -> Merge29/2
  GmG2kcaMcuCfgPer1/11(MotCtrlAdc0ScanGroup2Ref1) -> Merge31/2
  Merge32/1 -> Adc1ScanGroup3Ref0/1
  GmG2kcaMcuCfgInit3/1(Adc1ScanGroup3Ref0) -> Merge32/1
  GmG2kcaMcuCfgInit3/5(Adc1ScanGroup2Ref0) -> Merge34/1
  GmG2kcaMcuCfgInit3/4(Adc1ScanGroup3Ref1) -> Merge33/1
  Merge34/1 -> Adc1ScanGroup2Ref0/1
  Merge33/1 -> Adc1ScanGroup3Ref1/1
  GmG2kcaMcuCfgInit3/7(Adc1ScanGroup2Ref1) -> Merge35/1
  Merge35/1 -> Adc1ScanGroup2Ref1/1
  GmG2kcaMcuCfgPer2/1(Adc1ScanGroup3Ref0) -> Merge32/2
  GmG2kcaMcuCfgPer2/4(Adc1ScanGroup3Ref1) -> Merge33/2
  GmG2kcaMcuCfgPer2/5(Adc1ScanGroup2Ref0) -> Merge34/2
  GmG2kcaMcuCfgPer2/7(Adc1ScanGroup2Ref1) -> Merge35/2

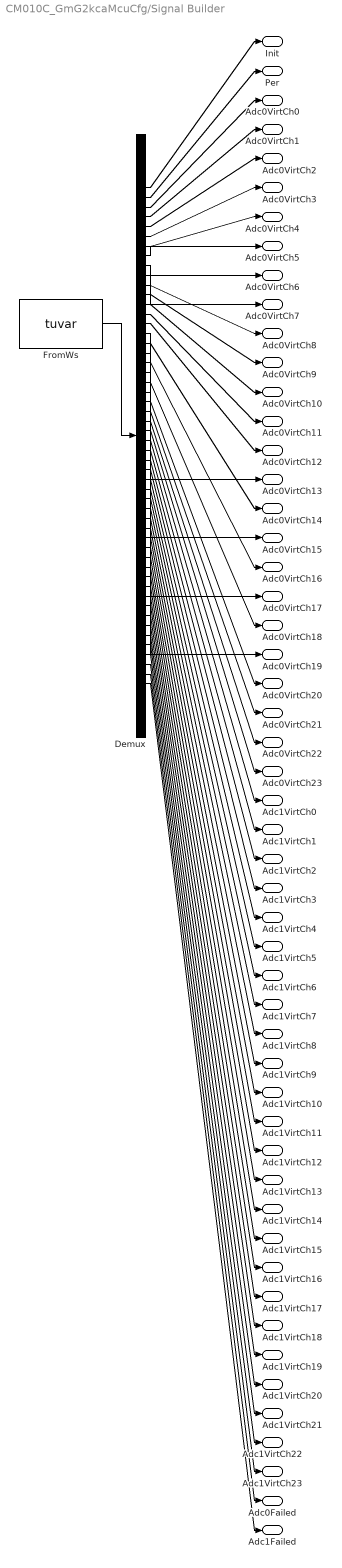
== system CM010C_GmG2kcaMcuCfg/Signal Builder ==
  Demux : Demux  Tag=STV Demux  Outputs=52
  FromWs : FromWorkspace  Tag=STV FromWs  VariableName=tuvar  SampleTime=0
      SigBuilderData=|
      | common.afterFinalStr = 'Extrapolate'
      | common.sampleTime = 0
      | dataSet.timeRange = [0 1]
      | dataSet.name = 'Sheet1'
      | sbobj.Name = 'Signal Builder'
      | sbobj.Groups.Name = 'Sheet1'
      | sbobj.Groups.Signals(1).Name = 'Init'
      | sbobj.Groups.Signals(1).XData = [0 0.001 0.001 1]
      | sbobj.Groups.Signals(1).YData = [1 1 0 0]
      | sbobj.Groups.Signals(2).Name = 'Per'
      | sbobj.Groups.Signals(2).XData = [0 0.001 0.001 1]
      | sbobj.Groups.Signals(2).YData = [0 0 1 1]
      | sbobj.Groups.Signals(3).Name = 'Adc0VirtCh0'
      | sbobj.Groups.Signals(3).XData = [0 1]
      | sbobj.Groups.Signals(3).YData = [0.72 0.72]
      | sbobj.Groups.Signals(4).Name = 'Adc0VirtCh1'
      | sbobj.Groups.Signals(4).XData = [0 0.002 0.004 0.006 0.008 0.01 1]
      | sbobj.Groups.Signals(4).YData = [1 1 1 1 1 1 1]
      | sbobj.Groups.Signals(5).Name = 'Adc0VirtCh2'
      | sbobj.Groups.Signals(5).XData = [0 0.002 0.004 0.006 0.008 0.01 1]
      | sbobj.Groups.Signals(5).YData = [1 1 1 1 1 1 1]
      | sbobj.Groups.Signals(6).Name = 'Adc0VirtCh3'
      | sbobj.Groups.Signals(6).XData = [0 0.002 0.004 0.006 0.008 0.01 1]
      | sbobj.Groups.Signals(6).YData = [1 1 1 1 1 1 1]
      | sbobj.Groups.Signals(7).Name = 'Adc0VirtCh4'
      | sbobj.Groups.Signals(7).XData = [0 0.002 0.004 0.006 0.008 0.01 1]
      | sbobj.Groups.Signals(7).YData = [1 1 1 1 1 1 1]
      | sbobj.Groups.Signals(8).Name = 'Adc0VirtCh5'
      | sbobj.Groups.Signals(8).XData = [0 0.002 0.004 0.006 0.008 0.01 1]
      | sbobj.Groups.Signals(8).YData = [1 1 1 1 1 1 1]
      | sbobj.Groups.Signals(9).Name = 'Adc0VirtCh6'
      | sbobj.Groups.Signals(9).XData = [0 0.002 0.004 0.006 0.008 0.01 1]
      | sbobj.Groups.Signals(9).YData = [1 1 1 1 1 1 1]
      | sbobj.Groups.Signals(10).Name = 'Adc0VirtCh7'
      | sbobj.Groups.Signals(10).XData = [0 0.002 0.004 0.006 0.008 0.01 1]
      | sbobj.Groups.Signals(10).YData = [1 1 1 1 1 1 1]
      | sbobj.Groups.Signals(11).Name = 'Adc0VirtCh8'
      | sbobj.Groups.Signals(11).XData = [0 0.002 0.004 0.006 0.008 0.01 1]
      | sbobj.Groups.Signals(11).YData = [1 1 1 1 1 1 1]
      | sbobj.Groups.Signals(12).Name = 'Adc0VirtCh9'
      | sbobj.Groups.Signals(12).XData = [0 0.002 0.004 0.006 0.008 0.01 1]
      | sbobj.Groups.Signals(12).YData = [1 1 1 1 1 1 1]
      | sbobj.Groups.Signals(13).Name = 'Adc0VirtCh10'
      | sbobj.Groups.Signals(13).XData = [0 0.002 0.004 0.006 0.008 0.01 1]
      | sbobj.Groups.Signals(13).YData = [1 1 1 1 1 1 1]
      | sbobj.Groups.Signals(14).Name = 'Adc0VirtCh11'
      | sbobj.Groups.Signals(14).XData = [0 0.002 0.004 0.006 0.008 0.01 1]
      | sbobj.Groups.Signals(14).YData = [1 1 1 1 1 1 1]
      | sbobj.Groups.Signals(15).Name = 'Adc0VirtCh12'
      | sbobj.Groups.Signals(15).XData = [0 0.002 0.004 0.006 0.008 0.01 1]
      | sbobj.Groups.Signals(15).YData = [1 1 1 1 1 1 1]
      | sbobj.Groups.Signals(16).Name = 'Adc0VirtCh13'
      | sbobj.Groups.Signals(16).XData = [0 0.002 0.004 0.006 0.008 0.01 1]
      | sbobj.Groups.Signals(16).YData = [1 1 1 1 1 1 1]
      | sbobj.Groups.Signals(17).Name = 'Adc0VirtCh14'
      | sbobj.Groups.Signals(17).XData = [0 0.002 0.004 0.006 0.008 0.01 1]
      | sbobj.Groups.Signals(17).YData = [1 1 1 1 1 1 1]
      | sbobj.Groups.Signals(18).Name = 'Adc0VirtCh15'
      | sbobj.Groups.Signals(18).XData = [0 0.002 0.004 0.006 0.008 0.01 1]
      | sbobj.Groups.Signals(18).YData = [1 1 1 1 1 1 1]
      | sbobj.Groups.Signals(19).Name = 'Adc0VirtCh16'
      | sbobj.Groups.Signals(19).XData = [0 0.002 0.004 0.006 0.008 0.01 1]
      | sbobj.Groups.Signals(19).YData = [1 1 1 1 1 1 1]
      | sbobj.Groups.Signals(20).Name = 'Adc0VirtCh17'
      | sbobj.Groups.Signals(20).XData = [0 0.002 0.004 0.006 0.008 0.01 1]
      | sbobj.Groups.Signals(20).YData = [1 1 1 1 1 1 1]
      | sbobj.Groups.Signals(21).Name = 'Adc0VirtCh18'
      | sbobj.Groups.Signals(21).XData = [0 0.002 0.004 0.006 0.008 0.01 1]
      | sbobj.Groups.Signals(21).YData = [1 1 1 1 1 1 1]
      | sbobj.Groups.Signals(22).Name = 'Adc0VirtCh19'
      | sbobj.Groups.Signals(22).XData = [0 0.002 0.004 0.006 0.008 0.01 1]
      | sbobj.Groups.Signals(22).YData = [1 1 1 1 1 1 1]
      | sbobj.Groups.Signals(23).Name = 'Adc0VirtCh20'
      | sbobj.Groups.Signals(23).XData = [0 0.002 0.004 0.006 0.008 0.01 1]
      | sbobj.Groups.Signals(23).YData = [1 1 1 1 1 1 1]
      | sbobj.Groups.Signals(24).Name = 'Adc0VirtCh21'
      | sbobj.Groups.Signals(24).XData = [0 0.002 0.004 0.006 0.008 0.01 1]
      | sbobj.Groups.Signals(24).YData = [1 1 1 1 1 1 1]
      | sbobj.Groups.Signals(25).Name = 'Adc0VirtCh22'
      | sbobj.Groups.Signals(25).XData = [0 0.002 0.004 0.006 0.008 0.01 1]
      | sbobj.Groups.Signals(25).YData = [1 1 1 1 1 1 1]
      | sbobj.Groups.Signals(26).Name = 'Adc0VirtCh23'
      | sbobj.Groups.Signals(26).XData = [0 0.002 0.004 0.006 0.008 0.01 1]
      | sbobj.Groups.Signals(26).YData = [1 1 1 1 1 1 1]
      | sbobj.Groups.Signals(27).Name = 'Adc1VirtCh0'
      | sbobj.Groups.Signals(27).XData = [0 0.002 0.004 0.006 0.008 0.01 1]
      | sbobj.Groups.Signals(27).YData = [1 1 1 1 1 1 1]
      | sbobj.Groups.Signals(28).Name = 'Adc1VirtCh1'
      | sbobj.Groups.Signals(28).XData = [0 0.002 0.004 0.006 0.008 0.01 1]
      | sbobj.Groups.Signals(28).YData = [1 1 1 1 1 1 1]
      | sbobj.Groups.Signals(29).Name = 'Adc1VirtCh2'
      | sbobj.Groups.Signals(29).XData = [0 0.002 0.004 0.006 0.008 0.01 1]
      | sbobj.Groups.Signals(29).YData = [1 1 1 1 1 1 1]
      | sbobj.Groups.Signals(30).Name = 'Adc1VirtCh3'
      | sbobj.Groups.Signals(30).XData = [0 0.002 0.004 0.006 0.008 0.01 1]
      | sbobj.Groups.Signals(30).YData = [1 1 1 1 1 1 1]
      | sbobj.Groups.Signals(31).Name = 'Adc1VirtCh4'
      | sbobj.Groups.Signals(31).XData = [0 0.002 0.004 0.006 0.008 0.01 1]
      | sbobj.Groups.Signals(31).YData = [1 1 1 1 1 1 1]
      | sbobj.Groups.Signals(32).Name = 'Adc1VirtCh5'
      | sbobj.Groups.Signals(32).XData = [0 0.010101010101 0.020202020202 0.030303030303 0.040404040404 0.0505050505051 0.0606060606061 0.0707070707071 0.0808080808081 0.0909090909091 0.10101010101 0.111111111111 0.121212121212 0.131313131313 0.141414141414 0.151515151515 0.161616161616 0.171717171717 0.181818181818 0.191919191919 0.20202020202 0.212121212121 0.222222222222 0.232323232323 0.242424242424 0.252525252525 0.262626262626 0.272727272727 0.282828282828 0.292929292929 0.30303030303 0.313131313131 0.323232323232 0.333333333333 0.343434343434 0.353535353535 0.363636363636 0.373737373737 0.383838383838 0.393939393939 0.40404040404 0.414141414141 0.424242424242 0.434343434343 0.444444444444 0.454545454545 0.464646464646 0.474747474747 0.484848484848 0.494949494949 0.505050505051 0.515151515152 0.525252525253 0.535353535354 0.545454545455 0.555555555556 0.565656565657 0.575757575758 0.585858585859 0.59595959596 0.606060606061 0.616161616162 0.626262626263 0.636363636364 0.646464646465 0.656565656566 0.666666666667 0.676767676768 0.686868686869 0.69696969697 0.707070707071 0.717171717172 0.727272727273 0.737373737374 0.747474747475 0.757575757576 0.767676767677 0.777777777778 0.787878787879 0.79797979798 0.808080808081 0.818181818182 0.828282828283 0.838383838384 0.848484848485 0.858585858586 0.868686868687 0.878787878788 0.888888888889 0.89898989899 0.909090909091 0.919191919192 0.929292929293 0.939393939394 0.949494949495 0.959595959596 0.969696969697 0.979797979798 0.989898989899 1]
      | sbobj.Groups.Signals(32).YData = [15 15.8879348752 16.77229435 17.649517421 18.5160718205 19.3684682398 20.2032743792 21.0171287692 21.8067543054 22.5689714444 23.3007110068 23.9990265356 24.6611061607 25.2842839212 25.8660505001 26.4040633287 26.8961560193 27.3403470883 27.734847935 28.0780700437 28.3686313802 28.6053619565 28.7873085422 28.9137385025 28.9841427486 28.9982377874 28.9559668633 28.8575001863 28.703234247 28.4937902198 28.230011462 27.9129601175 27.5439128401 27.124355653 26.6559779649 26.1406657674 25.580494041 24.9777183993 24.3347660072 23.6542258071 22.9388380941 22.191483482 21.4151713042 20.6130274957 19.7882820066 18.9442557958 18.084347459 17.2120195436 16.3307846063 15.444191069 14.555808931 13.6692153937 12.7879804564 11.915652541 11.0557442042 10.2117179934 9.38697250431 8.58482869582 7.80851651797 7.06116190592 6.34577419291 5.66523399277 5.0222816007 4.41950595904 3.85933423257 3.34402203511 2.87564434702 2.45608715992 2.08703988254 1.76998853799 1.50620978016 1.29676575299 1.14249981367 1.04403313667 1.00176221257 1.01585725144 1.08626149754 1.21269145783 1.39463804347 1.63136861978 1.92192995629 2.26515206504 2.65965291173 3.10384398071 3.5959366713 4.13394949992 4.71571607879 5.33889383925 6.00097346439 6.69928899324 7.43102855562 8.19324569459 8.98287123075 9.79672562076 10.6315317602 11.4839281795 12.350482579 13.22770565 14.1120651248 15]
      | sbobj.Groups.Signals(33).Name = 'Adc1VirtCh6'
      | sbobj.Groups.Signals(33).XData = [0 0.002 0.004 0.006 0.008 0.01 1]
      | sbobj.Groups.Signals(33).YData = [1 1 1 1 1 1 1]
      | sbobj.Groups.Signals(34).Name = 'Adc1VirtCh7'
      | sbobj.Groups.Signals(34).XData = [0 0.002 0.004 0.006 0.008 0.01 1]
      | sbobj.Groups.Signals(34).YData = [1 1 1 1 1 1 1]
      | sbobj.Groups.Signals(35).Name = 'Adc1VirtCh8'
      | sbobj.Groups.Signals(35).XData = [0 0.002 0.004 0.006 0.008 0.01 1]
      | sbobj.Groups.Signals(35).YData = [1 1 1 1 1 1 1]
      | sbobj.Groups.Signals(36).Name = 'Adc1VirtCh9'
      | sbobj.Groups.Signals(36).XData = [0 0.002 0.004 0.006 0.008 0.01 1]
      | sbobj.Groups.Signals(36).YData = [1 1 1 1 1 1 1]
      | sbobj.Groups.Signals(37).Name = 'Adc1VirtCh10'
      | sbobj.Groups.Signals(37).XData = [0 0.002 0.004 0.006 0.008 0.01 1]
      | sbobj.Groups.Signals(37).YData = [1 1 1 1 1 1 1]
      | sbobj.Groups.Signals(38).Name = 'Adc1VirtCh11'
      | sbobj.Groups.Signals(38).XData = [0 0.002 0.004 0.006 0.008 0.01 1]
      | sbobj.Groups.Signals(38).YData = [1 1 1 1 1 1 1]
      | sbobj.Groups.Signals(39).Name = 'Adc1VirtCh12'
      | sbobj.Groups.Signals(39).XData = [0 0.002 0.004 0.006 0.008 0.01 1]
      | sbobj.Groups.Signals(39).YData = [1 1 1 1 1 1 1]
      | sbobj.Groups.Signals(40).Name = 'Adc1VirtCh13'
      | sbobj.Groups.Signals(40).XData = [0 0.002 0.004 0.006 0.008 0.01 1]
      | sbobj.Groups.Signals(40).YData = [1 1 1 1 1 1 1]
      | sbobj.Groups.Signals(41).Name = 'Adc1VirtCh14'
      | sbobj.Groups.Signals(41).XData = [0 0.002 0.004 0.006 0.008 0.01 1]
      | sbobj.Groups.Signals(41).YData = [1 1 1 1 1 1 1]
      | sbobj.Groups.Signals(42).Name = 'Adc1VirtCh15'
      | sbobj.Groups.Signals(42).XData = [0 0.002 0.004 0.006 0.008 0.01 1]
      | sbobj.Groups.Signals(42).YData = [1 1 1 1 1 1 1]
      | sbobj.Groups.Signals(43).Name = 'Adc1VirtCh16'
      | sbobj.Groups.Signals(43).XData = [0 0.002 0.004 0.006 0.008 0.01 1]
      | sbobj.Groups.Signals(43).YData = [1 1 1 1 1 1 1]
      | sbobj.Groups.Signals(44).Name = 'Adc1VirtCh17'
      | sbobj.Groups.Signals(44).XData = [0 0.002 0.004 0.006 0.008 0.01 1]
      | sbobj.Groups.Signals(44).YData = [1 1 1 1 1 1 1]
      | sbobj.Groups.Signals(45).Name = 'Adc1VirtCh18'
      | sbobj.Groups.Signals(45).XData = [0 0.002 0.004 0.006 0.008 0.01 1]
      | sbobj.Groups.Signals(45).YData = [1 1 1 1 1 1 1]
      | sbobj.Groups.Signals(46).Name = 'Adc1VirtCh19'
      | sbobj.Groups.Signals(46).XData = [0 0.002 0.004 0.006 0.008 0.01 1]
      | sbobj.Groups.Signals(46).YData = [1 1 1 1 1 1 1]
      | sbobj.Groups.Signals(47).Name = 'Adc1VirtCh20'
      | sbobj.Groups.Signals(47).XData = [0 0.002 0.004 0.006 0.008 0.01 1]
      | sbobj.Groups.Signals(47).YData = [1 1 1 1 1 1 1]
      | sbobj.Groups.Signals(48).Name = 'Adc1VirtCh21'
      | sbobj.Groups.Signals(48).XData = [0 0.002 0.004 0.006 0.008 0.01 1]
      | sbobj.Groups.Signals(48).YData = [1 1 1 1 1 1 1]
      | sbobj.Groups.Signals(49).Name = 'Adc1VirtCh22'
      | sbobj.Groups.Signals(49).XData = [0 0.002 0.004 0.006 0.008 0.01 1]
      | sbobj.Groups.Signals(49).YData = [1 1 1 1 1 1 1]
      | sbobj.Groups.Signals(50).Name = 'Adc1VirtCh23'
      | sbobj.Groups.Signals(50).XData = [0 0.002 0.004 0.006 0.008 0.01 1]
      | sbobj.Groups.Signals(50).YData = [1 1 1 1 1 1 1]
      | sbobj.Groups.Signals(51).Name = 'Adc0Failed'
      | sbobj.Groups.Signals(51).XData = [0 0.886 0.886 0.898 0.898 1]
      | sbobj.Groups.Signals(51).YData = [0 0 1 1 0 0]
      | sbobj.Groups.Signals(52).Name = 'Adc1Failed'
      | sbobj.Groups.Signals(52).XData = [0 0.963 0.963 0.978 0.978 1]
      | sbobj.Groups.Signals(52).YData = [0 0 1 1 0 0]
      | sbobj.Groups.TimeRange = [0 1]
  Init : Outport
  Per : Outport  Tag=STV Outport  Port=2
  Adc0VirtCh0 : Outport  Tag=STV Outport  Port=3
  Adc0VirtCh1 : Outport  Tag=STV Outport  Port=4
  Adc0VirtCh2 : Outport  Tag=STV Outport  Port=5
  Adc0VirtCh3 : Outport  Tag=STV Outport  Port=6
  Adc0VirtCh4 : Outport  Tag=STV Outport  Port=7
  Adc0VirtCh5 : Outport  Tag=STV Outport  Port=8
  Adc0VirtCh6 : Outport  Tag=STV Outport  Port=9
  Adc0VirtCh7 : Outport  Tag=STV Outport  Port=10
  Adc0VirtCh8 : Outport  Tag=STV Outport  Port=11
  Adc0VirtCh9 : Outport  Tag=STV Outport  Port=12
  Adc0VirtCh10 : Outport  Tag=STV Outport  Port=13
  Adc0VirtCh11 : Outport  Tag=STV Outport  Port=14
  Adc0VirtCh12 : Outport  Tag=STV Outport  Port=15
  Adc0VirtCh13 : Outport  Tag=STV Outport  Port=16
  Adc0VirtCh14 : Outport  Tag=STV Outport  Port=17
  Adc0VirtCh15 : Outport  Tag=STV Outport  Port=18
  Adc0VirtCh16 : Outport  Tag=STV Outport  Port=19
  Adc0VirtCh17 : Outport  Tag=STV Outport  Port=20
  Adc0VirtCh18 : Outport  Tag=STV Outport  Port=21
  Adc0VirtCh19 : Outport  Tag=STV Outport  Port=22
  Adc0VirtCh20 : Outport  Tag=STV Outport  Port=23
  Adc0VirtCh21 : Outport  Tag=STV Outport  Port=24
  Adc0VirtCh22 : Outport  Tag=STV Outport  Port=25
  Adc0VirtCh23 : Outport  Tag=STV Outport  Port=26
  Adc1VirtCh0 : Outport  Tag=STV Outport  Port=27
  Adc1VirtCh1 : Outport  Tag=STV Outport  Port=28
  Adc1VirtCh2 : Outport  Tag=STV Outport  Port=29
  Adc1VirtCh3 : Outport  Tag=STV Outport  Port=30
  Adc1VirtCh4 : Outport  Tag=STV Outport  Port=31
  Adc1VirtCh5 : Outport  Tag=STV Outport  Port=32
  Adc1VirtCh6 : Outport  Tag=STV Outport  Port=33
  Adc1VirtCh7 : Outport  Tag=STV Outport  Port=34
  Adc1VirtCh8 : Outport  Tag=STV Outport  Port=35
  Adc1VirtCh9 : Outport  Tag=STV Outport  Port=36
  Adc1VirtCh10 : Outport  Tag=STV Outport  Port=37
  Adc1VirtCh11 : Outport  Tag=STV Outport  Port=38
  Adc1VirtCh12 : Outport  Tag=STV Outport  Port=39
  Adc1VirtCh13 : Outport  Tag=STV Outport  Port=40
  Adc1VirtCh14 : Outport  Tag=STV Outport  Port=41
  Adc1VirtCh15 : Outport  Tag=STV Outport  Port=42
  Adc1VirtCh16 : Outport  Tag=STV Outport  Port=43
  Adc1VirtCh17 : Outport  Tag=STV Outport  Port=44
  Adc1VirtCh18 : Outport  Tag=STV Outport  Port=45
  Adc1VirtCh19 : Outport  Tag=STV Outport  Port=46
  Adc1VirtCh20 : Outport  Tag=STV Outport  Port=47
  Adc1VirtCh21 : Outport  Tag=STV Outport  Port=48
  Adc1VirtCh22 : Outport  Tag=STV Outport  Port=49
  Adc1VirtCh23 : Outport  Tag=STV Outport  Port=50
  Adc0Failed : Outport  Tag=STV Outport  Port=51
  Adc1Failed : Outport  Tag=STV Outport  Port=52
  wires:
  FromWs/1 -> Demux/1
  Demux/1 -> Init/1
  Demux/2 -> Per/1
  Demux/3 -> Adc0VirtCh0/1
  Demux/4 -> Adc0VirtCh1/1
  Demux/5 -> Adc0VirtCh2/1
  Demux/6 -> Adc0VirtCh3/1
  Demux/7 -> Adc0VirtCh4/1
  Demux/8 -> Adc0VirtCh5/1
  Demux/9 -> Adc0VirtCh6/1
  Demux/10 -> Adc0VirtCh7/1
  Demux/11 -> Adc0VirtCh8/1
  Demux/12 -> Adc0VirtCh9/1
  Demux/13 -> Adc0VirtCh10/1
  Demux/14 -> Adc0VirtCh11/1
  Demux/15 -> Adc0VirtCh12/1
  Demux/16 -> Adc0VirtCh13/1
  Demux/17 -> Adc0VirtCh14/1
  Demux/18 -> Adc0VirtCh15/1
  Demux/19 -> Adc0VirtCh16/1
  Demux/20 -> Adc0VirtCh17/1
  Demux/21 -> Adc0VirtCh18/1
  Demux/22 -> Adc0VirtCh19/1
  Demux/23 -> Adc0VirtCh20/1
  Demux/24 -> Adc0VirtCh21/1
  Demux/25 -> Adc0VirtCh22/1
  Demux/26 -> Adc0VirtCh23/1
  Demux/27 -> Adc1VirtCh0/1
  Demux/28 -> Adc1VirtCh1/1
  Demux/29 -> Adc1VirtCh2/1
  Demux/30 -> Adc1VirtCh3/1
  Demux/31 -> Adc1VirtCh4/1
  Demux/32 -> Adc1VirtCh5/1
  Demux/33 -> Adc1VirtCh6/1
  Demux/34 -> Adc1VirtCh7/1
  Demux/35 -> Adc1VirtCh8/1
  Demux/36 -> Adc1VirtCh9/1
  Demux/37 -> Adc1VirtCh10/1
  Demux/38 -> Adc1VirtCh11/1
  Demux/39 -> Adc1VirtCh12/1
  Demux/40 -> Adc1VirtCh13/1
  Demux/41 -> Adc1VirtCh14/1
  Demux/42 -> Adc1VirtCh15/1
  Demux/43 -> Adc1VirtCh16/1
  Demux/44 -> Adc1VirtCh17/1
  Demux/45 -> Adc1VirtCh18/1
  Demux/46 -> Adc1VirtCh19/1
  Demux/47 -> Adc1VirtCh20/1
  Demux/48 -> Adc1VirtCh21/1
  Demux/49 -> Adc1VirtCh22/1
  Demux/50 -> Adc1VirtCh23/1
  Demux/51 -> Adc0Failed/1
  Demux/52 -> Adc1Failed/1

== system CM010C_GmG2kcaMcuCfg/GmG2kcaMcuCfg/CopyRight2 ==

== system CM010C_GmG2kcaMcuCfg/GmG2kcaMcuCfg/GmG2kcaMcuCfgInit1 ==
  function : TriggerPort  TriggerType=function-call
  CopyRight2 : Subsystem  Description=|  mask(Copyright Information){none=on}
      | Copyright info block.                                               
      |                                                                     
      | Place copyright information at the top of every subsystem in design.
      mask prompts: none "No parameters"
      mask help: Place copyright information at the top of every subsystem in design.
      mask Display:
      | NxtrConf = 'Nexteer Confidential';
      | 
      | sys = bdroot; %handle for the current model ("system")
      | first = get_param(sys,'Created');
      | first = first(end-3:end);  %year is last four digits
      | 
      | last = get_param(sys,'LastModifiedDate');
      | if isempty(last)
      |     last = datestr(now,'yyyy');
      | else
      |     last = last(end-3:end);
      | end
      | 
      | if strcmp(first,last)
      |     fprintf('%s -- Copyright %s Nexteer',NxtrConf,first)
      | else
      |     fprintf('%s -- %s%s- %s Nexteer',NxtrConf,char(169),first,last)
      | end
  Register Initialization : Subsystem  Priority=10
      settings: AttributesFormatString=Priority: %<Priority>

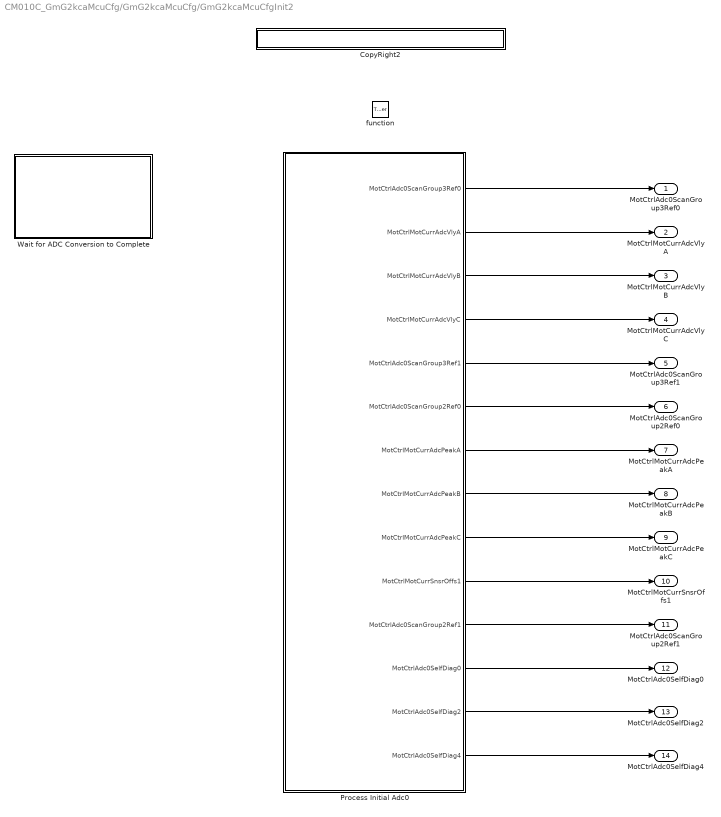
== system CM010C_GmG2kcaMcuCfg/GmG2kcaMcuCfg/GmG2kcaMcuCfgInit2 ==
  function : TriggerPort  TriggerType=function-call
  CopyRight2 : Subsystem  Description=|  mask(Copyright Information){none=on}
      | Copyright info block.                                               
      |                                                                     
      | Place copyright information at the top of every subsystem in design.
      mask prompts: none "No parameters"
      mask help: Place copyright information at the top of every subsystem in design.
      mask Display:
      | NxtrConf = 'Nexteer Confidential';
      | 
      | sys = bdroot; %handle for the current model ("system")
      | first = get_param(sys,'Created');
      | first = first(end-3:end);  %year is last four digits
      | 
      | last = get_param(sys,'LastModifiedDate');
      | if isempty(last)
      |     last = datestr(now,'yyyy');
      | else
      |     last = last(end-3:end);
      | end
      | 
      | if strcmp(first,last)
      |     fprintf('%s -- Copyright %s Nexteer',NxtrConf,first)
      | else
      |     fprintf('%s -- %s%s- %s Nexteer',NxtrConf,char(169),first,last)
      | end
  Process Initial Adc0 : Subsystem  RequirementInfo={} %GIDa_d862d82c_969a_40be_9cba_5dad28e4f649  Priority=20
      settings: AttributesFormatString=Priority: %<Priority>
  Wait for ADC Conversion to Complete : Subsystem  Priority=10
      settings: AttributesFormatString=Priority: %<Priority>
  MotCtrlAdc0ScanGroup3Ref0 : Outport
  MotCtrlMotCurrAdcVlyA : Outport  Port=2
  MotCtrlMotCurrAdcVlyB : Outport  Port=3
  MotCtrlMotCurrAdcVlyC : Outport  Port=4
  MotCtrlAdc0ScanGroup3Ref1 : Outport  Port=5
  MotCtrlAdc0ScanGroup2Ref0 : Outport  Port=6
  MotCtrlMotCurrAdcPeakA : Outport  Port=7
  MotCtrlMotCurrAdcPeakB : Outport  Port=8
  MotCtrlMotCurrAdcPeakC : Outport  Port=9
  MotCtrlMotCurrSnsrOffs1 : Outport  Port=10
  MotCtrlAdc0ScanGroup2Ref1 : Outport  Port=11
  MotCtrlAdc0SelfDiag0 : Outport  Port=12
  MotCtrlAdc0SelfDiag2 : Outport  Port=13
  MotCtrlAdc0SelfDiag4 : Outport  Port=14
  wires:
  Process Initial Adc0/2(MotCtrlMotCurrAdcVlyA) -> MotCtrlMotCurrAdcVlyA/1
  Process Initial Adc0/3(MotCtrlMotCurrAdcVlyB) -> MotCtrlMotCurrAdcVlyB/1
  Process Initial Adc0/4(MotCtrlMotCurrAdcVlyC) -> MotCtrlMotCurrAdcVlyC/1
  Process Initial Adc0/7(MotCtrlMotCurrAdcPeakA) -> MotCtrlMotCurrAdcPeakA/1
  Process Initial Adc0/8(MotCtrlMotCurrAdcPeakB) -> MotCtrlMotCurrAdcPeakB/1
  Process Initial Adc0/9(MotCtrlMotCurrAdcPeakC) -> MotCtrlMotCurrAdcPeakC/1
  Process Initial Adc0/10(MotCtrlMotCurrSnsrOffs1) -> MotCtrlMotCurrSnsrOffs1/1
  Process Initial Adc0/12(MotCtrlAdc0SelfDiag0) -> MotCtrlAdc0SelfDiag0/1
  Process Initial Adc0/13(MotCtrlAdc0SelfDiag2) -> MotCtrlAdc0SelfDiag2/1
  Process Initial Adc0/14(MotCtrlAdc0SelfDiag4) -> MotCtrlAdc0SelfDiag4/1
  Process Initial Adc0/5(MotCtrlAdc0ScanGroup3Ref1) -> MotCtrlAdc0ScanGroup3Ref1/1
  Process Initial Adc0/6(MotCtrlAdc0ScanGroup2Ref0) -> MotCtrlAdc0ScanGroup2Ref0/1
  Process Initial Adc0/1(MotCtrlAdc0ScanGroup3Ref0) -> MotCtrlAdc0ScanGroup3Ref0/1
  Process Initial Adc0/11(MotCtrlAdc0ScanGroup2Ref1) -> MotCtrlAdc0ScanGroup2Ref1/1

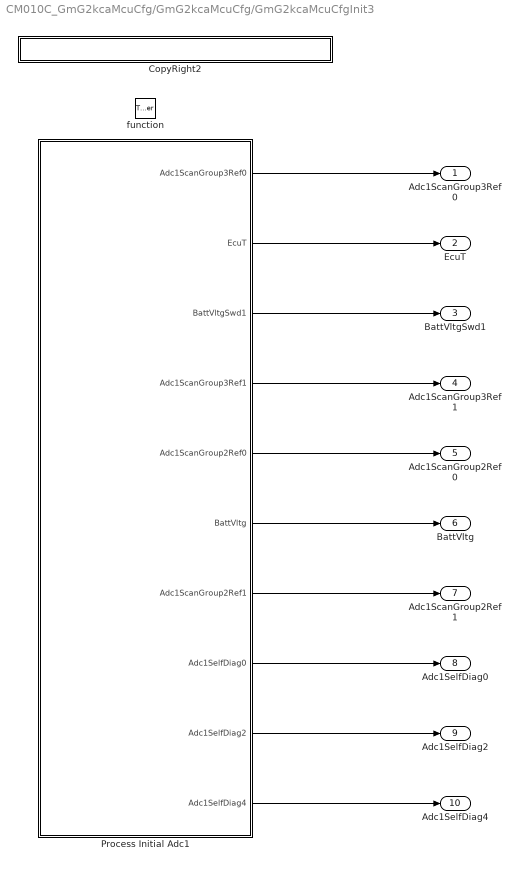
== system CM010C_GmG2kcaMcuCfg/GmG2kcaMcuCfg/GmG2kcaMcuCfgInit3 ==
  function : TriggerPort  TriggerType=function-call
  CopyRight2 : Subsystem  Description=|  mask(Copyright Information){none=on}
      | Copyright info block.                                               
      |                                                                     
      | Place copyright information at the top of every subsystem in design.
      mask prompts: none "No parameters"
      mask help: Place copyright information at the top of every subsystem in design.
      mask Display:
      | NxtrConf = 'Nexteer Confidential';
      | 
      | sys = bdroot; %handle for the current model ("system")
      | first = get_param(sys,'Created');
      | first = first(end-3:end);  %year is last four digits
      | 
      | last = get_param(sys,'LastModifiedDate');
      | if isempty(last)
      |     last = datestr(now,'yyyy');
      | else
      |     last = last(end-3:end);
      | end
      | 
      | if strcmp(first,last)
      |     fprintf('%s -- Copyright %s Nexteer',NxtrConf,first)
      | else
      |     fprintf('%s -- %s%s- %s Nexteer',NxtrConf,char(169),first,last)
      | end
  Process Initial Adc1 : Subsystem  RequirementInfo={} %GIDa_376048c3_94d2_40f9_9974_227dea3c5b4f  Priority=40
      settings: AttributesFormatString=Priority: %<Priority>
  Adc1ScanGroup3Ref0 : Outport
  EcuT : Outport  Port=2
  BattVltgSwd1 : Outport  Port=3
  Adc1ScanGroup3Ref1 : Outport  Port=4
  Adc1ScanGroup2Ref0 : Outport  Port=5
  BattVltg : Outport  Port=6
  Adc1ScanGroup2Ref1 : Outport  Port=7
  Adc1SelfDiag0 : Outport  Port=8
  Adc1SelfDiag2 : Outport  Port=9
  Adc1SelfDiag4 : Outport  Port=10
  wires:
  Process Initial Adc1/2(EcuT) -> EcuT/1
  Process Initial Adc1/3(BattVltgSwd1) -> BattVltgSwd1/1
  Process Initial Adc1/6(BattVltg) -> BattVltg/1
  Process Initial Adc1/8(Adc1SelfDiag0) -> Adc1SelfDiag0/1
  Process Initial Adc1/9(Adc1SelfDiag2) -> Adc1SelfDiag2/1
  Process Initial Adc1/10(Adc1SelfDiag4) -> Adc1SelfDiag4/1
  Process Initial Adc1/1(Adc1ScanGroup3Ref0) -> Adc1ScanGroup3Ref0/1
  Process Initial Adc1/4(Adc1ScanGroup3Ref1) -> Adc1ScanGroup3Ref1/1
  Process Initial Adc1/5(Adc1ScanGroup2Ref0) -> Adc1ScanGroup2Ref0/1
  Process Initial Adc1/7(Adc1ScanGroup2Ref1) -> Adc1ScanGroup2Ref1/1
